simulink library "initializeResponseSurface_cd"  (R2018a)
settings: Solver=VariableStepAuto  StartTime=0.0  StopTime=10.0  RelTol=1e-3
libraries: createRegressorMatrix x1, leastSquaresSolution_ul x1, storePerformanceIndex x1
settings Model: Creator=mitch  LastModifiedBy=mitch

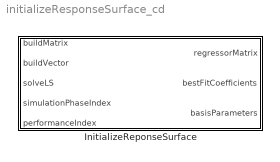
== system initializeResponseSurface_cd ==
  InitializeReponseSurface : Subsystem

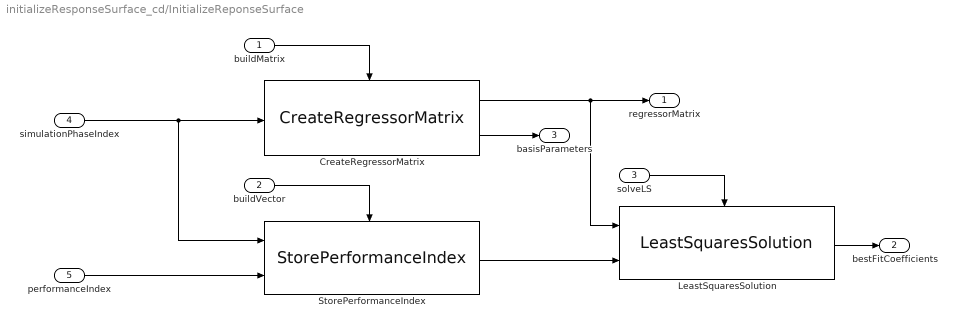
== system initializeResponseSurface_cd/InitializeReponseSurface ==
  buildMatrix : Inport
  buildVector : Inport  Port=2
  solveLS : Inport  Port=3
  simulationPhaseIndex : Inport  Port=4
  performanceIndex : Inport  Port=5
  CreateRegressorMatrix : createRegressorMatrix/CreateRegressorMatrix
  LeastSquaresSolution : leastSquaresSolution_ul/LeastSquaresSolution
  StorePerformanceIndex : storePerformanceIndex/StorePerformanceIndex
  regressorMatrix : Outport
  bestFitCoefficients : Outport  Port=2
  basisParameters : Outport  Port=3
  wires:
  simulationPhaseIndex/1 -> CreateRegressorMatrix/1, StorePerformanceIndex/1
  CreateRegressorMatrix/2 -> basisParameters/1
  CreateRegressorMatrix/1 -> regressorMatrix/1, LeastSquaresSolution/1
  StorePerformanceIndex/1 -> LeastSquaresSolution/2
  performanceIndex/1 -> StorePerformanceIndex/2
  LeastSquaresSolution/1 -> bestFitCoefficients/1
  buildMatrix/1 -> CreateRegressorMatrix/Enable
  solveLS/1 -> LeastSquaresSolution/Enable
  buildVector/1 -> StorePerformanceIndex/Enable
